simulink model "Backstepping_PSMC"  (Simulink 9.3)
settings: Solver=ode4  StartTime=0  StopTime=20.0  FixedStep=0.001  RelTol=1e-3  AbsTol=1e-6
libraries: Solver_SF x1
settings Model: Creator=ywata  LastModifiedBy=Dell Precision  ExtModeTrigMode=oneshot  ExtModeArmWhenConnect=off
settings SolverCC: AutoScaleAbsTol=off
settings DataIOCC: SignalLoggingName=sigsOut
settings OptimizationCC: BlockReduction=off  BooleanDataType=off
settings DebuggingCC: SaveWithParameterizedLinksMsg=none  SignalResolutionControl=TryResolveAllWithWarning  MultiTaskDSMMsg=warning  MultiTaskCondExecSysMsg=none  StateNameClashWarn=warning
settings HardwareCC: TargetUnknown=on
settings RTWCC: TemplateMakefile=grt_vc.tmf
settings GRTTargetCC: TargetFcnLib=ansi_tfl_tmw.mat  GeneratePreprocessorConditionals=Disable all

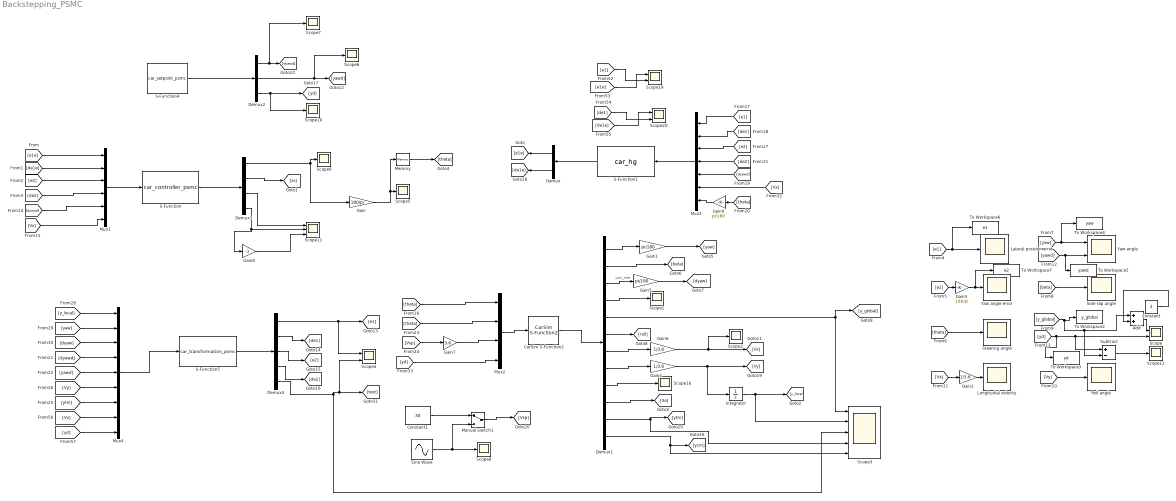
== system Backstepping_PSMC ==
  Add : Sum
  CarSim S-Function2 : Solver_SF/CarSim S-Function2  Priority=1  VehicleCode=i_i  SIMFILE=simfile.sim
      settings: AttributesFormatString=Vehicle Code: %<VehicleCode>
  Constant : Constant  Value=2
  Constant1 : Constant  Value=30
  Demux : Demux  Outputs=2
  Demux1 : Demux  Outputs=12
  Demux2 : Demux  Outputs=3
  Demux3 : Demux
  Demux4 : Demux  Outputs=5
  Gain : Gain  Gain=180/pi
  Gain1 : Gain  Gain=pi/180
  Gain2 : Gain  Gain=1/3.6
  Gain3 : Gain  Gain=180/pi
  Gain4 : Gain  Gain=1/3.6
  Gain5 : Gain  Gain=pi/180
  Gain6 : Gain  Gain=1/3.6
  Gain7 : Gain  Gain=3.6
  Gain8 : Gain  Gain=-1
  Gain9 : Gain  Gain=pi/180
  Integrator : Integrator
  Lateral posision error : Scope
  Longitudial velocity : Scope
  Manual Switch1 : ManualSwitch
  Memory : Memory
  Mux1 : Mux  Inputs=6
  Mux2 : Mux
  Mux3 : Mux  Inputs=7
  Mux4 : Mux  Inputs=9
  Roll angle : Scope
  S-Function : S-Function  FunctionName=car_controller_psmc  SFunctionDeploymentMode=off  EnableBusSupport=off
  S-Function1 : S-Function  FunctionName=car_hg  SFunctionDeploymentMode=off  EnableBusSupport=off
  S-Function4 : S-Function  FunctionName=car_setpoint_psmc  SFunctionDeploymentMode=off  EnableBusSupport=off
  S-Function5 : S-Function  FunctionName=car_transformation_psmc  SFunctionDeploymentMode=off  EnableBusSupport=off
  Scope{,4,19..20} (4 alike) : Scope  NumInputPorts=2
  Scope{1..2,5..10,12,16} (10 alike) : Scope
  Scope11 : Scope  NumInputPorts=3
  Scope3 : Scope  NumInputPorts=5
  Side slip angle : Scope
  Sine Wave : Sin  Amplitude=2  Bias=30  Frequency=0.5  SampleTime=0
  Steering angle : Scope
  Subtract : Sum  Inputs=+-
  To Workspace2 : ToWorkspace  VariableName=y_global  SaveFormat=Timeseries  SampleTime=-1
  To Workspace3 : ToWorkspace  VariableName=yd  SaveFormat=Timeseries  SampleTime=-1
  To Workspace4 : ToWorkspace  VariableName=yaw  SaveFormat=Timeseries  SampleTime=-1
  To Workspace5 : ToWorkspace  VariableName=yawd  SaveFormat=Timeseries  SampleTime=-1
  To Workspace6 : ToWorkspace  VariableName=e1  SaveFormat=Timeseries  SampleTime=-1
  To Workspace7 : ToWorkspace  VariableName=e2  SaveFormat=Timeseries  SampleTime=-1
  Yaw angle : Scope  NumInputPorts=2
  Yaw angle error : Scope
  wires:
  Demux2/3 -> Scope10/1, [yd]
  [dyaw] -> Mux4/3
  Demux4/1 -> [e1], Scope4/1
  [y_local] -> Mux4/1
  [de1e] -> Mux1/2
  Demux2/1 -> Scope7/1, [dyawd]
  Demux4/4 -> [de2]
  [de2] -> Mux1/4
  [e2] -> Gain3/1
  Demux4/2 -> [de1]
  [Vy] -> Roll angle/1
  Demux1/7 -> Gain6/1
  [yawd] -> To Workspace5/1, Yaw angle/2
  [theta] -> Steering angle/1
  Demux4/3 -> [e2]
  Gain1/1 -> [yaw]
  [yaw] -> Mux4/2
  Gain5/1 -> [dyaw]
  Gain/1 -> Memory/1, Scope5/1
  Gain2/1 -> Longitudial velocity/1
  [e2] -> Mux1/3
  [yawd] -> Mux4/5
  CarSim S-Function2/1 -> Demux1/1
  [e1e] -> Mux1/1
  [Vx] -> Gain2/1
  [e1] -> To Workspace6/1, Lateral posision error/1
  Demux1/6 -> [roll]
  [dyawd] -> Mux4/4
  Demux1/1 -> Gain1/1
  [beta] -> Side slip angle/1
  Demux1/8 -> Gain4/1
  [yaw] -> To Workspace4/1, Yaw angle/1
  Demux1/4 -> Scope1/1
  [yd] -> To Workspace3/1, Subtract/1, Scope/2
  Demux1/2 -> [beta]
  Demux1/5 -> [y_global], Scope3/1
  Demux1/3 -> Gain5/1  "yaw_rate"
  S-Function4/1 -> Demux2/1
  Demux3/1 -> Gain/1, Scope9/1
  Demux1/9 -> Scope16/1
  Demux1/10 -> [Xo]
  [Vsp] -> Gain7/1
  S-Function/1 -> Demux3/1
  Demux2/2 -> Scope6/1, [yawd]
  Sine Wave/1 -> Scope8/1, Manual Switch1/2
  Constant1/1 -> Manual Switch1/1
  Manual Switch1/1 -> [Vsp]
  Demux3/3 -> Scope11/1
  Demux3/4 -> Scope11/2, Gain8/1
  Gain8/1 -> Scope11/3
  Demux3/2 -> [ss]
  Subtract/1 -> Scope12/1
  [dyawd] -> Mux1/5
  Mux3/1 -> S-Function1/1
  [theta] -> Gain9/1
  [dyawd] -> Mux3/5
  [e1] -> Mux3/1
  [e2] -> Mux3/3
  [de2] -> Mux3/4
  [de1] -> Mux3/2
  Gain9/1 -> Mux3/7
  S-Function1/1 -> Demux/1
  Demux/2 -> [de1e]
  Demux/1 -> [e1e]
  [Vx] -> Mux3/6
  [de1] -> Scope20/2
  [de1e] -> Scope20/1
  [e1e] -> Scope19/1
  [e1] -> Scope19/2
  [y_global] -> To Workspace2/1, Subtract/2, Add/1
  Gain3/1 -> To Workspace7/1, Yaw angle error/1
  Mux2/1 -> CarSim S-Function2/1
  S-Function5/1 -> Demux4/1
  Gain7/1 -> Mux2/3
  [theta] -> Mux2/1
  [theta] -> Mux2/2
  [Vx] -> Mux1/6
  Mux4/1 -> S-Function5/1
  Gain6/1 -> Scope2/1, [Vx]
  Gain4/1 -> Integrator/1, [Vy]
  Mux1/1 -> S-Function/1
  [Vy] -> Mux4/6
  Integrator/1 -> Scope3/2, [y_local]
  [ytm] -> Mux4/7
  Demux1/11 -> [ytm], Scope3/4
  Demux1/12 -> Scope3/5, [ycm]
  Demux4/5 -> Scope3/3, [test], Scope4/2
  [Vx] -> Mux4/8
  [yd] -> Mux4/9
  Memory/1 -> [theta]
  [yd] -> Mux2/4
  Add/1 -> Scope/1
  Constant/1 -> Add/2
